simulink model "dspace_2019"  (R2019b)
settings: Solver=FixedStepDiscrete  StartTime=0.0  StopTime=Inf  FixedStep=1e-3  RelTol=1e-3
PostLoadFcn:
  | , if any(exist('dsrtsu_mdlpostloadfcn', 'file') ~= 0), dsrtsu_mdlpostloadfcn('Execute', bdroot); end,
undefined symbols (not defined in the file): ami, amk1_setpoints_1, amk2_setpoints_1, amk3_setpoints_1, amk4_setpoints_1, as, digital, ebs, indicator, mcu_set_dbu_indicator_points, mcu_set_ecu_indicator_points, res_ntm_node_control
libraries: rtican x63, simulink x5, rti1401lib_dio_type3 x4, simulink_extras x1
(part 8 of 16)

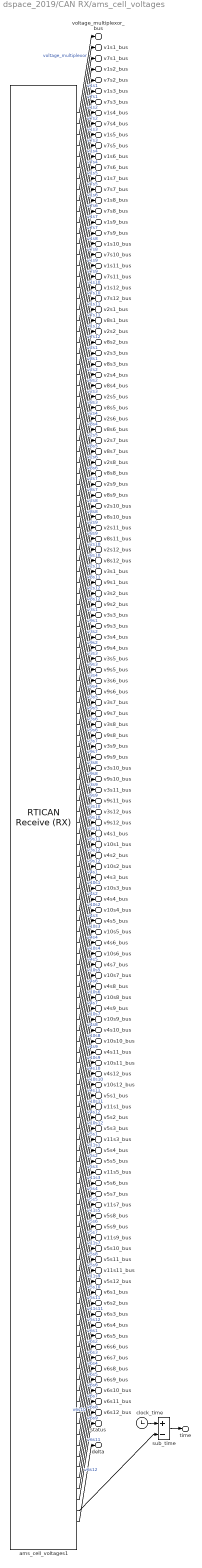
== system dspace_2019/CAN RX/ams_cell_voltages ==
  ams_cell_voltages1 : rtican/RTICAN Receive (RX)   Reserved1=[]  Reserved2=[]  Reserved3=[]  Reserved4=[]  SfcnMessage=[]  Msg_Struct=[]  BoardTypeNo=[]  BoardNo=[]  ChannelNo=[]  Parameters=[]  DialogFcn=[]  UnitName=[]  Revision=[]  UnitValues=[]  DSProperties=struct('RTI',struct('Version',uint32(5),'BlockType',struct('isSLSource',uint8(1),'isSLSink',uint8(1),'isHWSource',uint8(0),'isHWSink',uint8(0),'isSetup',uint8(0),'isInline',uint8(1),'isNonInline',uint8(0),'isInterrupt',uint8(0),'isChannelwise',uint8(0)),'IOBoardType','RTICAN','UnitType','MESSAGE','Identifier','RX','DialogType','MSVC','BlockSet','RTICAN','SlaveProcessor','CAN'))  RTIBlockInterface=struct('OutputPortsWidth',int32([1 1 1 1 1 1 1 1 1 1 1 1 1 1 1 1 1 1 1 1 1 1 1 1 1 1 1 1 1 1 1 1 1 1 1 1 1 1 1 1 1 1 1 1 1 1 1 1 1 1 1 1 1 1 1 1 1 1 1 1 1 1 1 1 1 1 1 1 1 1 1 1 1 1 1 1 1 1 1 1 1 1 1 1 1 1 1 1 1 1 1 1 1 1 1 1 1 1 1 1 1 1 1 1 1 1 1 1 1 1 1 1 1 1 1 1 1 1 1 1 1 1 1 1 1 1 1 1 1 1]),'OutputPortsActive',ones(1,130),'OutputPortsName',{{'voltage_multiplexor','v1s1','v7s1','v1s2','v7s2','v1s3','v7s3','v1s4','v7s4','v1s5','v7s5','v1s6','v7s6','v1s7','v7s7','v1s8','v7s8','v1s9','v7s9','v1s10','v7s10','v1s11','v7s11','v1s12','v7s12','v2s1','v8s1','v2s2','v8s2','v2s3','v8s3','v2s4','v8s4','v2s5','v8s5','v2s6','v8s6','v2s7','v8s7','v2s8','v8s8','v2s9','v8s9','v2s10','v8s10','v2s11','v8s11','v2s12','v8s12','v3s1','v9s1','v3s2','v9s2','v3s3','v9s3','v3s4','v9s4','v3s5','v9s5','v3s6','v9s6','v3s7','v9s7','v3s8','v9s8','v3s9','v9s9','v3s10','v9s10','v3s11','v9s11','v3s12','v9s12','v4s1','v10s1','v4s2','v10s2','v4s3','v10s3','v4s4','v10s4','v4s5','v10s5','v4s6','v10s6','v4s7','v10s7','v4s8','v10s8','v4s9','v10s9','v4s10','v10s10','v4s11','v10s11','v4s12','v10s12','v5s1','v11s1','v5s2','v5s3','v11s3','v5s4','v5s5','v11s5','v5s6','v5s7','v11s7','v5s8','v5s9','v11s9','v5s10','v5s11','v11s11','v5s12','v6s1','v6s2','v6s3','v6s4','v6s5','v6s6','v6s7','v6s8','v6s9','v6s10','v6s11','v6s12',['RX status'],['RX time'],['RX delta time']}},'OutputPortsDataType',{{'SS_DOUBLE','SS_DOUBLE','SS_DOUBLE','SS_DOUBLE','SS_DOUBLE','SS_DOUBLE','SS_DOUBLE','SS_DOUBLE','SS_DOUBLE','SS_DOUBLE','SS_DOUBLE','SS_DOUBLE','SS_DOUBLE','SS_DOUBLE','SS_DOUBLE','SS_DOUBLE','SS_DOUBLE','SS_DOUBLE','SS_DOUBLE','SS_DOUBLE','SS_DOUBLE','SS_DOUBLE','SS_DOUBLE','SS_DOUBLE','SS_DOUBLE','SS_DOUBLE','SS_DOUBLE','SS_DOUBLE','SS_DOUBLE','SS_DOUBLE','SS_DOUBLE','SS_DOUBLE','SS_DOUBLE','SS_DOUBLE','SS_DOUBLE','SS_DOUBLE','SS_DOUBLE','SS_DOUBLE','SS_DOUBLE','SS_DOUBLE','SS_DOUBLE','SS_DOUBLE','SS_DOUBLE','SS_DOUBLE','SS_DOUBLE','SS_DOUBLE','SS_DOUBLE','SS_DOUBLE','SS_DOUBLE','SS_DOUBLE','SS_DOUBLE','SS_DOUBLE','SS_DOUBLE','SS_DOUBLE','SS_DOUBLE','SS_DOUBLE','SS_DOUBLE','SS_DOUBLE','SS_DOUBLE','SS_DOUBLE','SS_DOUBLE','SS_DOUBLE','SS_DOUBLE','SS_DOUBLE','SS_DOUBLE','SS_DOUBLE','SS_DOUBLE','SS_DOUBLE','SS_DOUBLE','SS_DOUBLE','SS_DOUBLE','SS_DOUBLE','SS_DOUBLE','SS_DOUBLE','SS_DOUBLE','SS_DOUBLE','SS_DOUBLE','SS_DOUBLE','SS_DOUBLE','SS_DOUBLE','SS_DOUBLE','SS_DOUBLE','SS_DOUBLE','SS_DOUBLE','SS_DOUBLE','SS_DOUBLE','SS_DOUBLE','SS_DOUBLE','SS_DOUBLE','SS_DOUBLE','SS_DOUBLE','SS_DOUBLE','SS_DOUBLE','SS_DOUBLE','SS_DOUBLE','SS_DOUBLE','SS_DOUBLE','SS_DOUBLE','SS_DOUBLE','SS_DOUBLE','SS_DOUBLE','SS_DOUBLE','SS_DOUBLE','SS_DOUBLE','SS_DOUBLE','SS_DOUBLE','SS_DOUBLE','SS_DOUBLE','SS_DOUBLE','SS_DOUBLE','SS_DOUBLE','SS_DOUBLE','SS_DOUBLE','SS_DOUBLE','SS_DOUBLE','SS_DOUBLE','SS_DOUBLE','SS_DOUBLE','SS_DOUBLE','SS_DOUBLE','SS_DOUBLE','SS_DOUBLE','SS_DOUBLE','SS_DOUBLE','SS_DOUBLE','SS_DOUBLE','SS_DOUBLE','SS_DOUBLE','SS_DOUBLE','SS_DOUBLE'}},'OutputPortsLabel',{{'voltage_multiplexor','v1s1','v7s1','v1s2','v7s2','v1s3','v7s3','v1s4','v7s4','v1s5','v7s5','v1s6','v7s6','v1s7','v7s7','v1s8','v7s8','v1s9','v7s9','v1s10','v7s10','v1s11','v7s11','v1s12','v7s12','v2s1','v8s1','v2s2','v8s2','v2s3','v8s3','v2s4','v8s4','v2s5','v8s5','v2s6','v8s6','v2s7','v8s7','v2s8','v8s8','v2s9','v8s9','v2s10','v8s10','v2s11','v8s11','v2s12','v8s12','v3s1','v9s1','v3s2','v9s2','v3s3','v9s3','v3s4','v9s4','v3s5','v9s5','v3s6','v9s6','v3s7','v9s7','v3s8','v9s8','v3s9','v9s9','v3s10','v9s10','v3s11','v9s11','v3s12','v9s12','v4s1','v10s1','v4s2','v10s2','v4s3','v10s3','v4s4','v10s4','v4s5','v10s5','v4s6','v10s6','v4s7','v10s7','v4s8','v10s8','v4s9','v10s9','v4s10','v10s10','v4s11','v10s11','v4s12','v10s12','v5s1','v11s1','v5s2','v5s3','v11s3','v5s4','v5s5','v11s5','v5s6','v5s7','v11s7','v5s8','v5s9','v11s9','v5s10','v5s11','v11s11','v5s12','v6s1','v6s2','v6s3','v6s4','v6s5','v6s6','v6s7','v6s8','v6s9','v6s10','v6s11','v6s12','','',''}},'OutputPortsLabelMode','ON','InputPortsWidth',int32(0),'InputPortsActive',0,'DialogFcn','rtican_message_interface_gui','BlockDisplay',{{'','center'}},'IconTransparency','on','ParameterTunableNames',{{}},'InitLevel',3,'BlockName',struct('Token',{{'ams_cell_voltages'}}),'SampleTime',{{-1}},'TriggerPort',{{'none'}},'EnablePort',{{'none'}})  RTIBlockParameters=struct('BoardTypeNo',{{1,'OFF',[]}},'BoardNo',{{1,'ON',[1 16]}},'ChannelNo',{{2,'ON',[1 2]}},'Parameters',{{struct('DataFileSupport',struct('DataFileSelectedMaster',1,'DataFileSelectedLocal',1,'DataFileName','c:\users\oscar\documents\github\sw_infrastructure\kthfspe_python\databases\can1.dbc|','DataFileDate',{{{['10-Jul-2022 16:14:04']}}},'SelectedFile','c:\users\oscar\documents\github\sw_infrastructure\kthfspe_python\databases\can1.dbc'),'Options',struct('StatusSelected',1,'TimeSelected',1,'DeltaTimeSelected',1,'BytePortSelected',0,'MessageLengthSelected',0,'TriggerPort',struct('Selected',0,'TriggerType',0),'UserCoding',struct('Selected',0,'InterfaceFile','UserDecodingFile','FcnName','UserDecodeFcn','InportSelected',0,'InportWidth',1,'OutportSelected',0,'OutportWidth',1),'EnablePortSelected',0,'SignalOnPortnameSelected',1,'UseRXService',0),'Message',struct('MsgOnBlocknameSelected',1,'MsgName','ams_cell_voltages','MsgIdFormat',0,'MsgId',33,'MsgLength',7,'NumSignals',127,'SampleTime',-1,'Signal',struct('SgnName',{'voltage_multiplexor','v1s1','v7s1','v1s2','v7s2','v1s3','v7s3','v1s4','v7s4','v1s5','v7s5','v1s6','v7s6','v1s7','v7s7','v1s8','v7s8','v1s9','v7s9','v1s10','v7s10','v1s11','v7s11','v1s12','v7s12','v2s1','v8s1','v2s2','v8s2','v2s3','v8s3','v2s4','v8s4','v2s5','v8s5','v2s6','v8s6','v2s7','v8s7','v2s8','v8s8','v2s9','v8s9','v2s10','v8s10','v2s11','v8s11','v2s12','v8s12','v3s1','v9s1','v3s2','v9s2','v3s3','v9s3','v3s4','v9s4','v3s5','v9s5','v3s6','v9s6','v3s7','v9s7','v3s8','v9s8','v3s9','v9s9','v3s10','v9s10','v3s11','v9s11','v3s12','v9s12','v4s1','v10s1','v4s2','v10s2','v4s3','v10s3','v4s4','v10s4','v4s5','v10s5','v4s6','v10s6','v4s7','v10s7','v4s8','v10s8','v4s9','v10s9','v4s10','v10s10','v4s11','v10s11','v4s12','v10s12','v5s1','v11s1','v5s2','v5s3','v11s3','v5s4','v5s5','v11s5','v5s6','v5s7','v11s7','v5s8','v5s9','v11s9','v5s10','v5s11','v11s11','v5s12','v6s1','v6s2','v6s3','v6s4','v6s5','v6s6','v6s7','v6s8','v6s9','v6s10','v6s11','v6s12'},'SgnStartBit',{0,8,8,8,8,8,8,8,8,8,8,8,8,8,8,8,8,8,8,8,8,8,8,8,8,16,16,16,16,16,16,16,16,16,16,16,16,16,16,16,16,16,16,16,16,16,16,16,16,24,24,24,24,24,24,24,24,24,24,24,24,24,24,24,24,24,24,24,24,24,24,24,24,32,32,32,32,32,32,32,32,32,32,32,32,32,32,32,32,32,32,32,32,32,32,32,32,40,40,40,40,40,40,40,40,40,40,40,40,40,40,40,40,40,40,48,48,48,48,48,48,48,48,48,48,48,48},'SgnLength',{8,8,8,8,8,8,8,8,8,8,8,8,8,8,8,8,8,8,8,8,8,8,8,8,8,8,8,8,8,8,8,8,8,8,8,8,8,8,8,8,8,8,8,8,8,8,8,8,8,8,8,8,8,8,8,8,8,8,8,8,8,8,8,8,8,8,8,8,8,8,8,8,8,8,8,8,8,8,8,8,8,8,8,8,8,8,8,8,8,8,8,8,8,8,8,8,8,8,8,8,8,8,8,8,8,8,8,8,8,8,8,8,8,8,8,8,8,8,8,8,8,8,8,8,8,8,8},'SgnType',{1,2,2,2,2,2,2,2,2,2,2,2,2,2,2,2,2,2,2,2,2,2,2,2,2,2,2,2,2,2,2,2,2,2,2,2,2,2,2,2,2,2,2,2,2,2,2,2,2,2,2,2,2,2,2,2,2,2,2,2,2,2,2,2,2,2,2,2,2,2,2,2,2,2,2,2,2,2,2,2,2,2,2,2,2,2,2,2,2,2,2,2,2,2,2,2,2,2,2,2,2,2,2,2,2,2,2,2,2,2,2,2,2,2,2,2,2,2,2,2,2,2,2,2,2,2,2},'ModeValue',{-1,0,1,2,3,4,5,6,7,8,9,10,11,12,13,14,15,16,17,18,19,20,21,22,23,0,1,2,3,4,5,6,7,8,9,10,11,12,13,14,15,16,17,18,19,20,21,22,23,0,1,2,3,4,5,6,7,8,9,10,11,12,13,14,15,16,17,18,19,20,21,22,23,0,1,2,3,4,5,6,7,8,9,10,11,12,13,14,15,16,17,18,19,20,21,22,23,0,1,2,4,5,6,8,9,10,12,13,14,16,17,18,20,21,22,0,2,4,6,8,10,12,14,16,18,20,22},'DataType',{0,0,0,0,0,0,0,0,0,0,0,0,0,0,0,0,0,0,0,0,0,0,0,0,0,0,0,0,0,0,0,0,0,0,0,0,0,0,0,0,0,0,0,0,0,0,0,0,0,0,0,0,0,0,0,0,0,0,0,0,0,0,0,0,0,0,0,0,0,0,0,0,0,0,0,0,0,0,0,0,0,0,0,0,0,0,0,0,0,0,0,0,0,0,0,0,0,0,0,0,0,0,0,0,0,0,0,0,0,0,0,0,0,0,0,0,0,0,0,0,0,0,0,0,0,0,0},'ByteLayout',{0,0,0,0,0,0,0,0,0,0,0,0,0,0,0,0,0,0,0,0,0,0,0,0,0,0,0,0,0,0,0,0,0,0,0,0,0,0,0,0,0,0,0,0,0,0,0,0,0,0,0,0,0,0,0,0,0,0,0,0,0,0,0,0,0,0,0,0,0,0,0,0,0,0,0,0,0,0,0,0,0,0,0,0,0,0,0,0,0,0,0,0,0,0,0,0,0,0,0,0,0,0,0,0,0,0,0,0,0,0,0,0,0,0,0,0,0,0,0,0,0,0,0,0,0,0,0},'Factor',{1,0.00784,0.00784,0.00784,0.00784,0.00784,0.00784,0.00784,0.00784,0.00784,0.00784,0.00784,0.00784,0.00784,0.00784,0.00784,0.00784,0.00784,0.00784,0.00784,0.00784,0.00784,0.00784,0.00784,0.00784,0.00784,0.00784,0.00784,0.00784,0.00784,0.00784,0.00784,0.00784,0.00784,0.00784,0.00784,0.00784,0.00784,0.00784,0.00784,0.00784,0.00784,0.00784,0.00784,0.00784,0.00784,0.00784,0.00784,0.00784,0.00784,0.00784,0.00784,0.00784,0.00784,0.00784,0.00784,0.00784,0.00784,0.00784,0.00784,0.00784,0.00784,0.00784,0.00784,0.00784,0.00784,0.00784,0.00784,0.00784,0.00784,0.00784,0.00784,0.00784,0.00784,0.00784,0.00784,0.00784,0.00784,0.00784,0.00784,0.00784,0.00784,0.00784,0.00784,0.00784,0.00784,0.00784,0.00784,0.00784,0.00784,0.00784,0.00784,0.00784,0.00784,0.00784,0.00784,0.00784,0.00784,0.00784,0.00784,0.00784,0.00784,0.00784,0.00784,0.00784,0.00784,0.00784,0.00784,0.00784,0.00784,0.00784,0.00784,0.00784,0.00784,0.00784,0.00784,0.00784,0.00784,0.00784,0.00784,0.00784,0.00784,0.00784,0.00784,0.00784,0.00784,0.00784},'Offset',{0,2.5,2.5,2.5,2.5,2.5,2.5,2.5,2.5,2.5,2.5,2.5,2.5,2.5,2.5,2.5,2.5,2.5,2.5,2.5,2.5,2.5,2.5,2.5,2.5,2.5,2.5,2.5,2.5,2.5,2.5,2.5,2.5,2.5,2.5,2.5,2.5,2.5,2.5,2.5,2.5,2.5,2.5,2.5,2.5,2.5,2.5,2.5,2.5,2.5,2.5,2.5,2.5,2.5,2.5,2.5,2.5,2.5,2.5,2.5,2.5,2.5,2.5,2.5,2.5,2.5,2.5,2.5,2.5,2.5,2.5,2.5,2.5,2.5,2.5,2.5,2.5,2.5,2.5,2.5,2.5,2.5,2.5,2.5,2.5,2.5,2.5,2.5,2.5,2.5,2.5,2.5,2.5,2.5,2.5,2.5,2.5,2.5,2.5,2.5,2.5,2.5,2.5,2.5,2.5,2.5,2.5,2.5,2.5,2.5,2.5,2.5,2.5,2.5,2.5,2.5,2.5,2.5,2.5,2.5,2.5,2.5,2.5,2.5,2.5,2.5,2.5},'SgnComment',{{''},{''},{''},{''},{''},{''},{''},{''},{''},{''},{''},{''},{''},{''},{''},{''},{''},{''},{''},{''},{''},{''},{''},{''},{''},{''},{''},{''},{''},{''},{''},{''},{''},{''},{''},{''},{''},{''},{''},{''},{''},{''},{''},{''},{''},{''},{''},{''},{''},{''},{''},{''},{''},{''},{''},{''},{''},{''},{''},{''},{''},{''},{''},{''},{''},{''},{''},{''},{''},{''},{''},{''},{''},{''},{''},{''},{''},{''},{''},{''},{''},{''},{''},{''},{''},{''},{''},{''},{''},{''},{''},{''},{''},{''},{''},{''},{''},{''},{''},{''},{''},{''},{''},{''},{''},{''},{''},{''},{''},{''},{''},{''},{''},{''},{''},{''},{''},{''},{''},{''},{''},{''},{''},{''},{''},{''},{''}},'SgnUnit',{'','V','V','V','V','V','V','V','V','V','V','V','V','V','V','V','V','V','V','V','V','V','V','V','V','V','V','V','V','V','V','V','V','V','V','V','V','V','V','V','V','V','V','V','V','V','V','V','V','V','V','V','V','V','V','V','V','V','V','V','V','V','V','V','V','V','V','V','V','V','V','V','V','V','V','V','V','V','V','V','V','V','V','V','V','V','V','V','V','V','V','V','V','V','V','V','V','V','V','V','V','V','V','V','V','V','V','V','V','V','V','V','V','V','V','V','V','V','V','V','V','V','V','V','V','V','V'},'Min',{0,2.5,2.5,2.5,2.5,2.5,2.5,2.5,2.5,2.5,2.5,2.5,2.5,2.5,2.5,2.5,2.5,2.5,2.5,2.5,2.5,2.5,2.5,2.5,2.5,2.5,2.5,2.5,2.5,2.5,2.5,2.5,2.5,2.5,2.5,2.5,2.5,2.5,2.5,2.5,2.5,2.5,2.5,2.5,2.5,2.5,2.5,2.5,2.5,2.5,2.5,2.5,2.5,2.5,2.5,2.5,2.5,2.5,2.5,2.5,2.5,2.5,2.5,2.5,2.5,2.5,2.5,2.5,2.5,2.5,2.5,2.5,2.5,2.5,2.5,2.5,2.5,2.5,2.5,2.5,2.5,2.5,2.5,2.5,2.5,2.5,2.5,2.5,2.5,2.5,2.5,2.5,2.5,2.5,2.5,2.5,2.5,2.5,2.5,2.5,2.5,2.5,2.5,2.5,2.5,2.5,2.5,2.5,2.5,2.5,2.5,2.5,2.5,2.5,2.5,2.5,2.5,2.5,2.5,2.5,2.5,2.5,2.5,2.5,2.5,2.5,2.5},'Max',{0,4.5,4.5,4.5,4.5,4.5,4.5,4.5,4.5,4.5,4.5,4.5,4.5,4.5,4.5,4.5,4.5,4.5,4.5,4.5,4.5,4.5,4.5,4.5,4.5,4.5,4.5,4.5,4.5,4.5,4.5,4.5,4.5,4.5,4.5,4.5,4.5,4.5,4.5,4.5,4.5,4.5,4.5,4.5,4.5,4.5,4.5,4.5,4.5,4.5,4.5,4.5,4.5,4.5,4.5,4.5,4.5,4.5,4.5,4.5,4.5,4.5,4.5,4.5,4.5,4.5,4.5,4.5,4.5,4.5,4.5,4.5,4.5,4.5,4.5,4.5,4.5,4.5,4.5,4.5,4.5,4.5,4.5,4.5,4.5,4.5,4.5,4.5,4.5,4.5,4.5,4.5,4.5,4.5,4.5,4.5,4.5,4.5,4.5,4.5,4.5,4.5,4.5,4.5,4.5,4.5,4.5,4.5,4.5,4.5,4.5,4.5,4.5,4.5,4.5,4.5,4.5,4.5,4.5,4.5,4.5,4.5,4.5,4.5,4.5,4.5,4.5},'SLDataType',{'SS_DOUBLE','SS_DOUBLE','SS_DOUBLE','SS_DOUBLE','SS_DOUBLE','SS_DOUBLE','SS_DOUBLE','SS_DOUBLE','SS_DOUBLE','SS_DOUBLE','SS_DOUBLE','SS_DOUBLE','SS_DOUBLE','SS_DOUBLE','SS_DOUBLE','SS_DOUBLE','SS_DOUBLE','SS_DOUBLE','SS_DOUBLE','SS_DOUBLE','SS_DOUBLE','SS_DOUBLE','SS_DOUBLE','SS_DOUBLE','SS_DOUBLE','SS_DOUBLE','SS_DOUBLE','SS_DOUBLE','SS_DOUBLE','SS_DOUBLE','SS_DOUBLE','SS_DOUBLE','SS_DOUBLE','SS_DOUBLE','SS_DOUBLE','SS_DOUBLE','SS_DOUBLE','SS_DOUBLE','SS_DOUBLE','SS_DOUBLE','SS_DOUBLE','SS_DOUBLE','SS_DOUBLE','SS_DOUBLE','SS_DOUBLE','SS_DOUBLE','SS_DOUBLE','SS_DOUBLE','SS_DOUBLE','SS_DOUBLE','SS_DOUBLE','SS_DOUBLE','SS_DOUBLE','SS_DOUBLE','SS_DOUBLE','SS_DOUBLE','SS_DOUBLE','SS_DOUBLE','SS_DOUBLE','SS_DOUBLE','SS_DOUBLE','SS_DOUBLE','SS_DOUBLE','SS_DOUBLE','SS_DOUBLE','SS_DOUBLE','SS_DOUBLE','SS_DOUBLE','SS_DOUBLE','SS_DOUBLE','SS_DOUBLE','SS_DOUBLE','SS_DOUBLE','SS_DOUBLE','SS_DOUBLE','SS_DOUBLE','SS_DOUBLE','SS_DOUBLE','SS_DOUBLE','SS_DOUBLE','SS_DOUBLE','SS_DOUBLE','SS_DOUBLE','SS_DOUBLE','SS_DOUBLE','SS_DOUBLE','SS_DOUBLE','SS_DOUBLE','SS_DOUBLE','SS_DOUBLE','SS_DOUBLE','SS_DOUBLE','SS_DOUBLE','SS_DOUBLE','SS_DOUBLE','SS_DOUBLE','SS_DOUBLE','SS_DOUBLE','SS_DOUBLE','SS_DOUBLE','SS_DOUBLE','SS_DOUBLE','SS_DOUBLE','SS_DOUBLE','SS_DOUBLE','SS_DOUBLE','SS_DOUBLE','SS_DOUBLE','SS_DOUBLE','SS_DOUBLE','SS_DOUBLE','SS_DOUBLE','SS_DOUBLE','SS_DOUBLE','SS_DOUBLE','SS_DOUBLE','SS_DOUBLE','SS_DOUBLE','SS_DOUBLE','SS_DOUBLE','SS_DOUBLE','SS_DOUBLE','SS_DOUBLE','SS_DOUBLE','SS_DOUBLE','SS_DOUBLE','SS_DOUBLE'}),'MsgIdNumFormat',0,'MsgComment',{{''}}),'Version',1.2,'general',struct('isFromLib',0)),'OFF',[]}},'GroupId',{{struct('Group',{{'RTICAN'}},'No',1,'Behavior',{{'NAMECHANGE'}},'BlockType',{{'SINK'}},'NameChangeFlag',0),'OFF',[]}},'SFcnRTICANMessage',{{struct('MsgType','RX','SFcnPortType','Scalar','MsgName','ams_cell_voltages','MsgIdFormat','STD','MsgId',33,'MsgLength',7,'NumSignals',127,'SampleTime',-1,'Signal',struct('SgnName',{'voltage_multiplexor','v1s1','v7s1','v1s2','v7s2','v1s3','v7s3','v1s4','v7s4','v1s5','v7s5','v1s6','v7s6','v1s7','v7s7','v1s8','v7s8','v1s9','v7s9','v1s10','v7s10','v1s11','v7s11','v1s12','v7s12','v2s1','v8s1','v2s2','v8s2','v2s3','v8s3','v2s4','v8s4','v2s5','v8s5','v2s6','v8s6','v2s7','v8s7','v2s8','v8s8','v2s9','v8s9','v2s10','v8s10','v2s11','v8s11','v2s12','v8s12','v3s1','v9s1','v3s2','v9s2','v3s3','v9s3','v3s4','v9s4','v3s5','v9s5','v3s6','v9s6','v3s7','v9s7','v3s8','v9s8','v3s9','v9s9','v3s10','v9s10','v3s11','v9s11','v3s12','v9s12','v4s1','v10s1','v4s2','v10s2','v4s3','v10s3','v4s4','v10s4','v4s5','v10s5','v4s6','v10s6','v4s7','v10s7','v4s8','v10s8','v4s9','v10s9','v4s10','v10s10','v4s11','v10s11','v4s12','v10s12','v5s1','v11s1','v5s2','v5s3','v11s3','v5s4','v5s5','v11s5','v5s6','v5s7','v11s7','v5s8','v5s9','v11s9','v5s10','v5s11','v11s11','v5s12','v6s1','v6s2','v6s3','v6s4','v6s5','v6s6','v6s7','v6s8','v6s9','v6s10','v6s11','v6s12'},'SgnStartBit',{0,8,8,8,8,8,8,8,8,8,8,8,8,8,8,8,8,8,8,8,8,8,8,8,8,16,16,16,16,16,16,16,16,16,16,16,16,16,16,16,16,16,16,16,16,16,16,16,16,24,24,24,24,24,24,24,24,24,24,24,24,24,24,24,24,24,24,24,24,24,24,24,24,32,32,32,32,32,32,32,32,32,32,32,32,32,32,32,32,32,32,32,32,32,32,32,32,40,40,40,40,40,40,40,40,40,40,40,40,40,40,40,40,40,40,48,48,48,48,48,48,48,48,48,48,48,48},'SgnLength',{8,8,8,8,8,8,8,8,8,8,8,8,8,8,8,8,8,8,8,8,8,8,8,8,8,8,8,8,8,8,8,8,8,8,8,8,8,8,8,8,8,8,8,8,8,8,8,8,8,8,8,8,8,8,8,8,8,8,8,8,8,8,8,8,8,8,8,8,8,8,8,8,8,8,8,8,8,8,8,8,8,8,8,8,8,8,8,8,8,8,8,8,8,8,8,8,8,8,8,8,8,8,8,8,8,8,8,8,8,8,8,8,8,8,8,8,8,8,8,8,8,8,8,8,8,8,8},'SgnType',{'mode','mode-dependent','mode-dependent','mode-dependent','mode-dependent','mode-dependent','mode-dependent','mode-dependent','mode-dependent','mode-dependent','mode-dependent','mode-dependent','mode-dependent','mode-dependent','mode-dependent','mode-dependent','mode-dependent','mode-dependent','mode-dependent','mode-dependent','mode-dependent','mode-dependent','mode-dependent','mode-dependent','mode-dependent','mode-dependent','mode-dependent','mode-dependent','mode-dependent','mode-dependent','mode-dependent','mode-dependent','mode-dependent','mode-dependent','mode-dependent','mode-dependent','mode-dependent','mode-dependent','mode-dependent','mode-dependent','mode-dependent','mode-dependent','mode-dependent','mode-dependent','mode-dependent','mode-dependent','mode-dependent','mode-dependent','mode-dependent','mode-dependent','mode-dependent','mode-dependent','mode-dependent','mode-dependent','mode-dependent','mode-dependent','mode-dependent','mode-dependent','mode-dependent','mode-dependent','mode-dependent','mode-dependent','mode-dependent','mode-dependent','mode-dependent','mode-dependent','mode-dependent','mode-dependent','mode-dependent','mode-dependent','mode-dependent','mode-dependent','mode-dependent','mode-dependent','mode-dependent','mode-dependent','mode-dependent','mode-dependent','mode-dependent','mode-dependent','mode-dependent','mode-dependent','mode-dependent','mode-dependent','mode-dependent','mode-dependent','mode-dependent','mode-dependent','mode-dependent','mode-dependent','mode-dependent','mode-dependent','mode-dependent','mode-dependent','mode-dependent','mode-dependent','mode-dependent','mode-dependent','mode-dependent','mode-dependent','mode-dependent','mode-dependent','mode-dependent','mode-dependent','mode-dependent','mode-dependent','mode-dependent','mode-dependent','mode-dependent','mode-dependent','mode-dependent','mode-dependent','mode-dependent','mode-dependent','mode-dependent','mode-dependent','mode-dependent','mode-dependent','mode-dependent','mode-dependent','mode-dependent','mode-dependent','mode-dependent','mode-dependent','mode-dependent','mode-dependent','mode-dependent'},'ModeValue',{-1,0,1,2,3,4,5,6,7,8,9,10,11,12,13,14,15,16,17,18,19,20,21,22,23,0,1,2,3,4,5,6,7,8,9,10,11,12,13,14,15,16,17,18,19,20,21,22,23,0,1,2,3,4,5,6,7,8,9,10,11,12,13,14,15,16,17,18,19,20,21,22,23,0,1,2,3,4,5,6,7,8,9,10,11,12,13,14,15,16,17,18,19,20,21,22,23,0,1,2,4,5,6,8,9,10,12,13,14,16,17,18,20,21,22,0,2,4,6,8,10,12,14,16,18,20,22},'DataType',{['unsigned int'],['unsigned int'],['unsigned int'],['unsigned int'],['unsigned int'],['unsigned int'],['unsigned int'],['unsigned int'],['unsigned int'],['unsigned int'],['unsigned int'],['unsigned int'],['unsigned int'],['unsigned int'],['unsigned int'],['unsigned int'],['unsigned int'],['unsigned int'],['unsigned int'],['unsigned int'],['unsigned int'],['unsigned int'],['unsigned int'],['unsigned int'],['unsigned int'],['unsigned int'],['unsigned int'],['unsigned int'],['unsigned int'],['unsigned int'],['unsigned int'],['unsigned int'],['unsigned int'],['unsigned int'],['unsigned int'],['unsigned int'],['unsigned int'],['unsigned int'],['unsigned int'],['unsigned int'],['unsigned int'],['unsigned int'],['unsigned int'],['unsigned int'],['unsigned int'],['unsigned int'],['unsigned int'],['unsigned int'],['unsigned int'],['unsigned int'],['unsigned int'],['unsigned int'],['unsigned int'],['unsigned int'],['unsigned int'],['unsigned int'],['unsigned int'],['unsigned int'],['unsigned int'],['unsigned int'],['unsigned int'],['unsigned int'],['unsigned int'],['unsigned int'],['unsigned int'],['unsigned int'],['unsigned int'],['unsigned int'],['unsigned int'],['unsigned int'],['unsigned int'],['unsigned int'],['unsigned int'],['unsigned int'],['unsigned int'],['unsigned int'],['unsigned int'],['unsigned int'],['unsigned int'],['unsigned int'],['unsigned int'],['unsigned int'],['unsigned int'],['unsigned int'],['unsigned int'],['unsigned int'],['unsigned int'],['unsigned int'],['unsigned int'],['unsigned int'],['unsigned int'],['unsigned int'],['unsigned int'],['unsigned int'],['unsigned int'],['unsigned int'],['unsigned int'],['unsigned int'],['unsigned int'],['unsigned int'],['unsigned int'],['unsigned int'],['unsigned int'],['unsigned int'],['unsigned int'],['unsigned int'],['unsigned int'],['unsigned int'],['unsigned int'],['unsigned int'],['unsigned int'],['unsigned int'],['unsigned int'],['unsigned int'],['unsigned int'],['unsigned int'],['unsigned int'],['unsigned int'],['unsigned int'],['unsigned int'],['unsigned int'],['unsigned int'],['unsigned int'],['unsigned int'],['unsigned int'],['unsigned int'],['unsigned int']},'ByteLayout',{['little endian'],['little endian'],['little endian'],['little endian'],['little endian'],['little endian'],['little endian'],['little endian'],['little endian'],['little endian'],['little endian'],['little endian'],['little endian'],['little endian'],['little endian'],['little endian'],['little endian'],['little endian'],['little endian'],['little endian'],['little endian'],['little endian'],['little endian'],['little endian'],['little endian'],['little endian'],['little endian'],['little endian'],['little endian'],['little endian'],['little endian'],['little endian'],['little endian'],['little endian'],['little endian'],['little endian'],['little endian'],['little endian'],['little endian'],['little endian'],['little endian'],['little endian'],['little endian'],['little endian'],['little endian'],['little endian'],['little endian'],['little endian'],['little endian'],['little endian'],['little endian'],['little endian'],['little endian'],['little endian'],['little endian'],['little endian'],['little endian'],['little endian'],['little endian'],['little endian'],['little endian'],['little endian'],['little endian'],['little endian'],['little endian'],['little endian'],['little endian'],['little endian'],['little endian'],['little endian'],['little endian'],['little endian'],['little endian'],['little endian'],['little endian'],['little endian'],['little endian'],['little endian'],['little endian'],['little endian'],['little endian'],['little endian'],['little endian'],['little endian'],['little endian'],['little endian'],['little endian'],['little endian'],['little endian'],['little endian'],['little endian'],['little endian'],['little endian'],['little endian'],['little endian'],['little endian'],['little endian'],['little endian'],['little endian'],['little endian'],['little endian'],['little endian'],['little endian'],['little endian'],['little endian'],['little endian'],['little endian'],['little endian'],['little endian'],['little endian'],['little endian'],['little endian'],['little endian'],['little endian'],['little endian'],['little endian'],['little endian'],['little endian'],['little endian'],['little endian'],['little endian'],['little endian'],['little endian'],['little endian'],['little endian'],['little endian'],['little endian']},'Factor',{1,0.00784,0.00784,0.00784,0.00784,0.00784,0.00784,0.00784,0.00784,0.00784,0.00784,0.00784,0.00784,0.00784,0.00784,0.00784,0.00784,0.00784,0.00784,0.00784,0.00784,0.00784,0.00784,0.00784,0.00784,0.00784,0.00784,0.00784,0.00784,0.00784,0.00784,0.00784,0.00784,0.00784,0.00784,0.00784,0.00784,0.00784,0.00784,0.00784,0.00784,0.00784,0.00784,0.00784,0.00784,0.00784,0.00784,0.00784,0.00784,0.00784,0.00784,0.00784,0.00784,0.00784,0.00784,0.00784,0.00784,0.00784,0.00784,0.00784,0.00784,0.00784,0.00784,0.00784,0.00784,0.00784,0.00784,0.00784,0.00784,0.00784,0.00784,0.00784,0.00784,0.00784,0.00784,0.00784,0.00784,0.00784,0.00784,0.00784,0.00784,0.00784,0.00784,0.00784,0.00784,0.00784,0.00784,0.00784,0.00784,0.00784,0.00784,0.00784,0.00784,0.00784,0.00784,0.00784,0.00784,0.00784,0.00784,0.00784,0.00784,0.00784,0.00784,0.00784,0.00784,0.00784,0.00784,0.00784,0.00784,0.00784,0.00784,0.00784,0.00784,0.00784,0.00784,0.00784,0.00784,0.00784,0.00784,0.00784,0.00784,0.00784,0.00784,0.00784,0.00784,0.00784,0.00784},'Offset',{0,2.5,2.5,2.5,2.5,2.5,2.5,2.5,2.5,2.5,2.5,2.5,2.5,2.5,2.5,2.5,2.5,2.5,2.5,2.5,2.5,2.5,2.5,2.5,2.5,2.5,2.5,2.5,2.5,2.5,2.5,2.5,2.5,2.5,2.5,2.5,2.5,2.5,2.5,2.5,2.5,2.5,2.5,2.5,2.5,2.5,2.5,2.5,2.5,2.5,2.5,2.5,2.5,2.5,2.5,2.5,2.5,2.5,2.5,2.5,2.5,2.5,2.5,2.5,2.5,2.5,2.5,2.5,2.5,2.5,2.5,2.5,2.5,2.5,2.5,2.5,2.5,2.5,2.5,2.5,2.5,2.5,2.5,2.5,2.5,2.5,2.5,2.5,2.5,2.5,2.5,2.5,2.5,2.5,2.5,2.5,2.5,2.5,2.5,2.5,2.5,2.5,2.5,2.5,2.5,2.5,2.5,2.5,2.5,2.5,2.5,2.5,2.5,2.5,2.5,2.5,2.5,2.5,2.5,2.5,2.5,2.5,2.5,2.5,2.5,2.5,2.5},'SLDataType',{'SS_DOUBLE','SS_DOUBLE','SS_DOUBLE','SS_DOUBLE','SS_DOUBLE','SS_DOUBLE','SS_DOUBLE','SS_DOUBLE','SS_DOUBLE','SS_DOUBLE','SS_DOUBLE','SS_DOUBLE','SS_DOUBLE','SS_DOUBLE','SS_DOUBLE','SS_DOUBLE','SS_DOUBLE','SS_DOUBLE','SS_DOUBLE','SS_DOUBLE','SS_DOUBLE','SS_DOUBLE','SS_DOUBLE','SS_DOUBLE','SS_DOUBLE','SS_DOUBLE','SS_DOUBLE','SS_DOUBLE','SS_DOUBLE','SS_DOUBLE','SS_DOUBLE','SS_DOUBLE','SS_DOUBLE','SS_DOUBLE','SS_DOUBLE','SS_DOUBLE','SS_DOUBLE','SS_DOUBLE','SS_DOUBLE','SS_DOUBLE','SS_DOUBLE','SS_DOUBLE','SS_DOUBLE','SS_DOUBLE','SS_DOUBLE','SS_DOUBLE','SS_DOUBLE','SS_DOUBLE','SS_DOUBLE','SS_DOUBLE','SS_DOUBLE','SS_DOUBLE','SS_DOUBLE','SS_DOUBLE','SS_DOUBLE','SS_DOUBLE','SS_DOUBLE','SS_DOUBLE','SS_DOUBLE','SS_DOUBLE','SS_DOUBLE','SS_DOUBLE','SS_DOUBLE','SS_DOUBLE','SS_DOUBLE','SS_DOUBLE','SS_DOUBLE','SS_DOUBLE','SS_DOUBLE','SS_DOUBLE','SS_DOUBLE','SS_DOUBLE','SS_DOUBLE','SS_DOUBLE','SS_DOUBLE','SS_DOUBLE','SS_DOUBLE','SS_DOUBLE','SS_DOUBLE','SS_DOUBLE','SS_DOUBLE','SS_DOUBLE','SS_DOUBLE','SS_DOUBLE','SS_DOUBLE','SS_DOUBLE','SS_DOUBLE','SS_DOUBLE','SS_DOUBLE','SS_DOUBLE','SS_DOUBLE','SS_DOUBLE','SS_DOUBLE','SS_DOUBLE','SS_DOUBLE','SS_DOUBLE','SS_DOUBLE','SS_DOUBLE','SS_DOUBLE','SS_DOUBLE','SS_DOUBLE','SS_DOUBLE','SS_DOUBLE','SS_DOUBLE','SS_DOUBLE','SS_DOUBLE','SS_DOUBLE','SS_DOUBLE','SS_DOUBLE','SS_DOUBLE','SS_DOUBLE','SS_DOUBLE','SS_DOUBLE','SS_DOUBLE','SS_DOUBLE','SS_DOUBLE','SS_DOUBLE','SS_DOUBLE','SS_DOUBLE','SS_DOUBLE','SS_DOUBLE','SS_DOUBLE','SS_DOUBLE','SS_DOUBLE','SS_DOUBLE','SS_DOUBLE','SS_DOUBLE'}),'StatusSelected','yes','TimeSelected','yes','DeltaTimeSelected','yes','BytePortSelected','no','MessageLengthSelected','no','TriggerPort',struct('Selected','no','TriggerType',0),'UserCoding',struct('Selected','no','InterfaceFile','UserDecodingFile','FcnName','UserDecodeFcn','InportSelected','no','InportWidth',1,'OutportSelected','no','OutportWidth',1),'EnablePortSelected','no','UseRXService','no','BoardType','DS1','BoardNo',1,'ControllerNo',1),'OFF',[]}},'TLCFileName',{{'rtican_rx_message','OFF',[]}})  RTISFcnParameters=struct('SFcnRTICANMessage','struct','TLCFileName','char')  RTIBlockParaDefault=struct('BoardTypeNo',4302,'BoardNo',1,'ChannelNo',1,'Parameters',struct('DataFileSupport',struct('DataFileSelectedMaster',0,'DataFileSelectedLocal',0,'DataFileName','','DataFileDate','','SelectedFile',['<no file selected>']),'Options',struct('StatusSelected',1,'TimeSelected',1,'DeltaTimeSelected',1,'BytePortSelected',0,'MessageLengthSelected',0,'TriggerPort',struct('Selected',0,'TriggerType','rising'),'UserCoding',struct('Selected',0,'InterfaceFile','UserDecodingFile','FcnName','UserDecodeFcn','InportSelected',0,'InportWidth',1,'OutportSelected',0,'OutportWidth',1),'EnablePortSelected',0,'SignalOnPortnameSelected',1,'UseRXService',0),'Message',struct('MsgOnBlocknameSelected',0,'MsgName',['RX Message'],'MsgIdFormat',0,'MsgId',100,'MsgLength',8,'NumSignals',1,'SampleTime',-1,'Signal',struct('SgnName',['RX signal'],'SgnStartBit',0,'SgnLength',8,'SgnType',0,'ModeValue',-1,'DataType',0,'SLDataType','SS_DOUBLE','ByteLayout',0,'Factor',1,'Offset',0,'Min',0,'Max',255,'SgnComment',{{}},'SgnUnit',''),'MsgIdNumFormat',0,'MsgComment',{{''}}),'Version',1.2,'general',struct('isFromLib',1)),'GroupId',struct('Group',{{'RTICAN'}},'No',1,'Behavior',{{'NAMECHANGE'}},'BlockType',{{'SINK'}},'NameChangeFlag',0),'SFcnRTICANMessage',struct('MsgType','RX','MsgName',['RX Message'],'MsgIdFormat','STD','MsgId',100,'MsgLength',8,'NumSignals',1,'SampleTime',-1,'Signal',struct('SgnName',['RX signal'],'SgnStartBit',0,'SgnLength',8,'SgnType','standard','ModeValue',-1,'DataType',['unsigned int'],'ByteLayout',['little endian'],'SLDataType','SS_DOUBLE','Factor',1,'Offset',0),'StatusSelected','yes','TimeSelected','yes','DeltaTimeSelected','yes','BytePortSelected','no','MessageLengthSelected','no','EnablePortSelected','no','UserCoding',struct('Selected','no','InterfaceFile','UserDecodingFile','FcnName','UserDecodeFcn','InportSelected','no','InportWidth',1,'OutportSelected','no','OutportWidth',1),'TriggerPort',struct('Selected','no','TriggerType','rising'),'UseRXService','no','BoardType','DS4302','BoardNo',1,'ControllerNo',1,'SFcnPortType','Scalar'),'TLCFileName','rtican_rx_message')
      settings: AttributesFormatString=Group Id: RTICAN1\n  SourceProductName=dSPACE RTI CAN Blockset
  clock_time : Clock
  sub_time : Sum  Inputs=+-
  voltage_multiplexor_bus : Outport  PortName=signals  Element=voltage_multiplexor
  v1s1_bus : Outport  PortName=signals  Element=v1s1
  v7s1_bus : Outport  PortName=signals  Element=v7s1
  v1s2_bus : Outport  PortName=signals  Element=v1s2
  v7s2_bus : Outport  PortName=signals  Element=v7s2
  v1s3_bus : Outport  PortName=signals  Element=v1s3
  v7s3_bus : Outport  PortName=signals  Element=v7s3
  v1s4_bus : Outport  PortName=signals  Element=v1s4
  v7s4_bus : Outport  PortName=signals  Element=v7s4
  v1s5_bus : Outport  PortName=signals  Element=v1s5
  v7s5_bus : Outport  PortName=signals  Element=v7s5
  v1s6_bus : Outport  PortName=signals  Element=v1s6
  v7s6_bus : Outport  PortName=signals  Element=v7s6
  v1s7_bus : Outport  PortName=signals  Element=v1s7
  v7s7_bus : Outport  PortName=signals  Element=v7s7
  v1s8_bus : Outport  PortName=signals  Element=v1s8
  v7s8_bus : Outport  PortName=signals  Element=v7s8
  v1s9_bus : Outport  PortName=signals  Element=v1s9
  v7s9_bus : Outport  PortName=signals  Element=v7s9
  v1s10_bus : Outport  PortName=signals  Element=v1s10
  v7s10_bus : Outport  PortName=signals  Element=v7s10
  v1s11_bus : Outport  PortName=signals  Element=v1s11
  v7s11_bus : Outport  PortName=signals  Element=v7s11
  v1s12_bus : Outport  PortName=signals  Element=v1s12
  v7s12_bus : Outport  PortName=signals  Element=v7s12
  v2s1_bus : Outport  PortName=signals  Element=v2s1
  v8s1_bus : Outport  PortName=signals  Element=v8s1
  v2s2_bus : Outport  PortName=signals  Element=v2s2
  v8s2_bus : Outport  PortName=signals  Element=v8s2
  v2s3_bus : Outport  PortName=signals  Element=v2s3
  v8s3_bus : Outport  PortName=signals  Element=v8s3
  v2s4_bus : Outport  PortName=signals  Element=v2s4
  v8s4_bus : Outport  PortName=signals  Element=v8s4
  v2s5_bus : Outport  PortName=signals  Element=v2s5
  v8s5_bus : Outport  PortName=signals  Element=v8s5
  v2s6_bus : Outport  PortName=signals  Element=v2s6
  v8s6_bus : Outport  PortName=signals  Element=v8s6
  v2s7_bus : Outport  PortName=signals  Element=v2s7
  v8s7_bus : Outport  PortName=signals  Element=v8s7
  v2s8_bus : Outport  PortName=signals  Element=v2s8
  v8s8_bus : Outport  PortName=signals  Element=v8s8
  v2s9_bus : Outport  PortName=signals  Element=v2s9
  v8s9_bus : Outport  PortName=signals  Element=v8s9
  v2s10_bus : Outport  PortName=signals  Element=v2s10
  v8s10_bus : Outport  PortName=signals  Element=v8s10
  v2s11_bus : Outport  PortName=signals  Element=v2s11
  v8s11_bus : Outport  PortName=signals  Element=v8s11
  v2s12_bus : Outport  PortName=signals  Element=v2s12
  v8s12_bus : Outport  PortName=signals  Element=v8s12
  v3s1_bus : Outport  PortName=signals  Element=v3s1
  v9s1_bus : Outport  PortName=signals  Element=v9s1
  v3s2_bus : Outport  PortName=signals  Element=v3s2
  v9s2_bus : Outport  PortName=signals  Element=v9s2
  v3s3_bus : Outport  PortName=signals  Element=v3s3
  v9s3_bus : Outport  PortName=signals  Element=v9s3
  v3s4_bus : Outport  PortName=signals  Element=v3s4
  v9s4_bus : Outport  PortName=signals  Element=v9s4
  v3s5_bus : Outport  PortName=signals  Element=v3s5
  v9s5_bus : Outport  PortName=signals  Element=v9s5
  v3s6_bus : Outport  PortName=signals  Element=v3s6
  v9s6_bus : Outport  PortName=signals  Element=v9s6
  v3s7_bus : Outport  PortName=signals  Element=v3s7
  v9s7_bus : Outport  PortName=signals  Element=v9s7
  v3s8_bus : Outport  PortName=signals  Element=v3s8
  v9s8_bus : Outport  PortName=signals  Element=v9s8
  v3s9_bus : Outport  PortName=signals  Element=v3s9
  v9s9_bus : Outport  PortName=signals  Element=v9s9
  v3s10_bus : Outport  PortName=signals  Element=v3s10
  v9s10_bus : Outport  PortName=signals  Element=v9s10
  v3s11_bus : Outport  PortName=signals  Element=v3s11
  v9s11_bus : Outport  PortName=signals  Element=v9s11
  v3s12_bus : Outport  PortName=signals  Element=v3s12
  v9s12_bus : Outport  PortName=signals  Element=v9s12
  v4s1_bus : Outport  PortName=signals  Element=v4s1
  v10s1_bus : Outport  PortName=signals  Element=v10s1
  v4s2_bus : Outport  PortName=signals  Element=v4s2
  v10s2_bus : Outport  PortName=signals  Element=v10s2
  v4s3_bus : Outport  PortName=signals  Element=v4s3
  v10s3_bus : Outport  PortName=signals  Element=v10s3
  v4s4_bus : Outport  PortName=signals  Element=v4s4
  v10s4_bus : Outport  PortName=signals  Element=v10s4
  v4s5_bus : Outport  PortName=signals  Element=v4s5
  v10s5_bus : Outport  PortName=signals  Element=v10s5
  v4s6_bus : Outport  PortName=signals  Element=v4s6
  v10s6_bus : Outport  PortName=signals  Element=v10s6
  v4s7_bus : Outport  PortName=signals  Element=v4s7
  v10s7_bus : Outport  PortName=signals  Element=v10s7
  v4s8_bus : Outport  PortName=signals  Element=v4s8
  v10s8_bus : Outport  PortName=signals  Element=v10s8
  v4s9_bus : Outport  PortName=signals  Element=v4s9
  v10s9_bus : Outport  PortName=signals  Element=v10s9
  v4s10_bus : Outport  PortName=signals  Element=v4s10
  v10s10_bus : Outport  PortName=signals  Element=v10s10
  v4s11_bus : Outport  PortName=signals  Element=v4s11
  v10s11_bus : Outport  PortName=signals  Element=v10s11
  v4s12_bus : Outport  PortName=signals  Element=v4s12
  v10s12_bus : Outport  PortName=signals  Element=v10s12
  v5s1_bus : Outport  PortName=signals  Element=v5s1
  v11s1_bus : Outport  PortName=signals  Element=v11s1
  v5s2_bus : Outport  PortName=signals  Element=v5s2
  v5s3_bus : Outport  PortName=signals  Element=v5s3
  v11s3_bus : Outport  PortName=signals  Element=v11s3
  v5s4_bus : Outport  PortName=signals  Element=v5s4
  v5s5_bus : Outport  PortName=signals  Element=v5s5
  v11s5_bus : Outport  PortName=signals  Element=v11s5
  v5s6_bus : Outport  PortName=signals  Element=v5s6
  v5s7_bus : Outport  PortName=signals  Element=v5s7
  v11s7_bus : Outport  PortName=signals  Element=v11s7
  v5s8_bus : Outport  PortName=signals  Element=v5s8
  v5s9_bus : Outport  PortName=signals  Element=v5s9
  v11s9_bus : Outport  PortName=signals  Element=v11s9
  v5s10_bus : Outport  PortName=signals  Element=v5s10
  v5s11_bus : Outport  PortName=signals  Element=v5s11
  v11s11_bus : Outport  PortName=signals  Element=v11s11
  v5s12_bus : Outport  PortName=signals  Element=v5s12
  v6s1_bus : Outport  PortName=signals  Element=v6s1
  v6s2_bus : Outport  PortName=signals  Element=v6s2
  v6s3_bus : Outport  PortName=signals  Element=v6s3
  v6s4_bus : Outport  PortName=signals  Element=v6s4
  v6s5_bus : Outport  PortName=signals  Element=v6s5
  v6s6_bus : Outport  PortName=signals  Element=v6s6
  v6s7_bus : Outport  PortName=signals  Element=v6s7
  v6s8_bus : Outport  PortName=signals  Element=v6s8
  v6s9_bus : Outport  PortName=signals  Element=v6s9
  v6s10_bus : Outport  PortName=signals  Element=v6s10
  v6s11_bus : Outport  PortName=signals  Element=v6s11
  v6s12_bus : Outport  PortName=signals  Element=v6s12
  status : Outport  Port=2
  time : Outport  Port=3
  delta : Outport  Port=4
  wires:
  clock_time/1 -> sub_time/1
  sub_time/1 -> time/1
  ams_cell_voltages1/128 -> status/1
  ams_cell_voltages1/129 -> sub_time/2
  ams_cell_voltages1/130 -> delta/1
  ams_cell_voltages1/1 -> voltage_multiplexor_bus/1  "voltage_multiplexor"
  ams_cell_voltages1/2 -> v1s1_bus/1  "v1s1"
  ams_cell_voltages1/3 -> v7s1_bus/1  "v7s1"
  ams_cell_voltages1/4 -> v1s2_bus/1  "v1s2"
  ams_cell_voltages1/5 -> v7s2_bus/1  "v7s2"
  ams_cell_voltages1/6 -> v1s3_bus/1  "v1s3"
  ams_cell_voltages1/7 -> v7s3_bus/1  "v7s3"
  ams_cell_voltages1/8 -> v1s4_bus/1  "v1s4"
  ams_cell_voltages1/9 -> v7s4_bus/1  "v7s4"
  ams_cell_voltages1/10 -> v1s5_bus/1  "v1s5"
  ams_cell_voltages1/11 -> v7s5_bus/1  "v7s5"
  ams_cell_voltages1/12 -> v1s6_bus/1  "v1s6"
  ams_cell_voltages1/13 -> v7s6_bus/1  "v7s6"
  ams_cell_voltages1/14 -> v1s7_bus/1  "v1s7"
  ams_cell_voltages1/15 -> v7s7_bus/1  "v7s7"
  ams_cell_voltages1/16 -> v1s8_bus/1  "v1s8"
  ams_cell_voltages1/17 -> v7s8_bus/1  "v7s8"
  ams_cell_voltages1/18 -> v1s9_bus/1  "v1s9"
  ams_cell_voltages1/19 -> v7s9_bus/1  "v7s9"
  ams_cell_voltages1/20 -> v1s10_bus/1  "v1s10"
  ams_cell_voltages1/21 -> v7s10_bus/1  "v7s10"
  ams_cell_voltages1/22 -> v1s11_bus/1  "v1s11"
  ams_cell_voltages1/23 -> v7s11_bus/1  "v7s11"
  ams_cell_voltages1/24 -> v1s12_bus/1  "v1s12"
  ams_cell_voltages1/25 -> v7s12_bus/1  "v7s12"
  ams_cell_voltages1/26 -> v2s1_bus/1  "v2s1"
  ams_cell_voltages1/27 -> v8s1_bus/1  "v8s1"
  ams_cell_voltages1/28 -> v2s2_bus/1  "v2s2"
  ams_cell_voltages1/29 -> v8s2_bus/1  "v8s2"
  ams_cell_voltages1/30 -> v2s3_bus/1  "v2s3"
  ams_cell_voltages1/31 -> v8s3_bus/1  "v8s3"
  ams_cell_voltages1/32 -> v2s4_bus/1  "v2s4"
  ams_cell_voltages1/33 -> v8s4_bus/1  "v8s4"
  ams_cell_voltages1/34 -> v2s5_bus/1  "v2s5"
  ams_cell_voltages1/35 -> v8s5_bus/1  "v8s5"
  ams_cell_voltages1/36 -> v2s6_bus/1  "v2s6"
  ams_cell_voltages1/37 -> v8s6_bus/1  "v8s6"
  ams_cell_voltages1/38 -> v2s7_bus/1  "v2s7"
  ams_cell_voltages1/39 -> v8s7_bus/1  "v8s7"
  ams_cell_voltages1/40 -> v2s8_bus/1  "v2s8"
  ams_cell_voltages1/41 -> v8s8_bus/1  "v8s8"
  ams_cell_voltages1/42 -> v2s9_bus/1  "v2s9"
  ams_cell_voltages1/43 -> v8s9_bus/1  "v8s9"
  ams_cell_voltages1/44 -> v2s10_bus/1  "v2s10"
  ams_cell_voltages1/45 -> v8s10_bus/1  "v8s10"
  ams_cell_voltages1/46 -> v2s11_bus/1  "v2s11"
  ams_cell_voltages1/47 -> v8s11_bus/1  "v8s11"
  ams_cell_voltages1/48 -> v2s12_bus/1  "v2s12"
  ams_cell_voltages1/49 -> v8s12_bus/1  "v8s12"
  ams_cell_voltages1/50 -> v3s1_bus/1  "v3s1"
  ams_cell_voltages1/51 -> v9s1_bus/1  "v9s1"
  ams_cell_voltages1/52 -> v3s2_bus/1  "v3s2"
  ams_cell_voltages1/53 -> v9s2_bus/1  "v9s2"
  ams_cell_voltages1/54 -> v3s3_bus/1  "v3s3"
  ams_cell_voltages1/55 -> v9s3_bus/1  "v9s3"
  ams_cell_voltages1/56 -> v3s4_bus/1  "v3s4"
  ams_cell_voltages1/57 -> v9s4_bus/1  "v9s4"
  ams_cell_voltages1/58 -> v3s5_bus/1  "v3s5"
  ams_cell_voltages1/59 -> v9s5_bus/1  "v9s5"
  ams_cell_voltages1/60 -> v3s6_bus/1  "v3s6"
  ams_cell_voltages1/61 -> v9s6_bus/1  "v9s6"
  ams_cell_voltages1/62 -> v3s7_bus/1  "v3s7"
  ams_cell_voltages1/63 -> v9s7_bus/1  "v9s7"
  ams_cell_voltages1/64 -> v3s8_bus/1  "v3s8"
  ams_cell_voltages1/65 -> v9s8_bus/1  "v9s8"
  ams_cell_voltages1/66 -> v3s9_bus/1  "v3s9"
  ams_cell_voltages1/67 -> v9s9_bus/1  "v9s9"
  ams_cell_voltages1/68 -> v3s10_bus/1  "v3s10"
  ams_cell_voltages1/69 -> v9s10_bus/1  "v9s10"
  ams_cell_voltages1/70 -> v3s11_bus/1  "v3s11"
  ams_cell_voltages1/71 -> v9s11_bus/1  "v9s11"
  ams_cell_voltages1/72 -> v3s12_bus/1  "v3s12"
  ams_cell_voltages1/73 -> v9s12_bus/1  "v9s12"
  ams_cell_voltages1/74 -> v4s1_bus/1  "v4s1"
  ams_cell_voltages1/75 -> v10s1_bus/1  "v10s1"
  ams_cell_voltages1/76 -> v4s2_bus/1  "v4s2"
  ams_cell_voltages1/77 -> v10s2_bus/1  "v10s2"
  ams_cell_voltages1/78 -> v4s3_bus/1  "v4s3"
  ams_cell_voltages1/79 -> v10s3_bus/1  "v10s3"
  ams_cell_voltages1/80 -> v4s4_bus/1  "v4s4"
  ams_cell_voltages1/81 -> v10s4_bus/1  "v10s4"
  ams_cell_voltages1/82 -> v4s5_bus/1  "v4s5"
  ams_cell_voltages1/83 -> v10s5_bus/1  "v10s5"
  ams_cell_voltages1/84 -> v4s6_bus/1  "v4s6"
  ams_cell_voltages1/85 -> v10s6_bus/1  "v10s6"
  ams_cell_voltages1/86 -> v4s7_bus/1  "v4s7"
  ams_cell_voltages1/87 -> v10s7_bus/1  "v10s7"
  ams_cell_voltages1/88 -> v4s8_bus/1  "v4s8"
  ams_cell_voltages1/89 -> v10s8_bus/1  "v10s8"
  ams_cell_voltages1/90 -> v4s9_bus/1  "v4s9"
  ams_cell_voltages1/91 -> v10s9_bus/1  "v10s9"
  ams_cell_voltages1/92 -> v4s10_bus/1  "v4s10"
  ams_cell_voltages1/93 -> v10s10_bus/1  "v10s10"
  ams_cell_voltages1/94 -> v4s11_bus/1  "v4s11"
  ams_cell_voltages1/95 -> v10s11_bus/1  "v10s11"
  ams_cell_voltages1/96 -> v4s12_bus/1  "v4s12"
  ams_cell_voltages1/97 -> v10s12_bus/1  "v10s12"
  ams_cell_voltages1/98 -> v5s1_bus/1  "v5s1"
  ams_cell_voltages1/99 -> v11s1_bus/1  "v11s1"
  ams_cell_voltages1/100 -> v5s2_bus/1  "v5s2"
  ams_cell_voltages1/101 -> v5s3_bus/1  "v5s3"
  ams_cell_voltages1/102 -> v11s3_bus/1  "v11s3"
  ams_cell_voltages1/103 -> v5s4_bus/1  "v5s4"
  ams_cell_voltages1/104 -> v5s5_bus/1  "v5s5"
  ams_cell_voltages1/105 -> v11s5_bus/1  "v11s5"
  ams_cell_voltages1/106 -> v5s6_bus/1  "v5s6"
  ams_cell_voltages1/107 -> v5s7_bus/1  "v5s7"
  ams_cell_voltages1/108 -> v11s7_bus/1  "v11s7"
  ams_cell_voltages1/109 -> v5s8_bus/1  "v5s8"
  ams_cell_voltages1/110 -> v5s9_bus/1  "v5s9"
  ams_cell_voltages1/111 -> v11s9_bus/1  "v11s9"
  ams_cell_voltages1/112 -> v5s10_bus/1  "v5s10"
  ams_cell_voltages1/113 -> v5s11_bus/1  "v5s11"
  ams_cell_voltages1/114 -> v11s11_bus/1  "v11s11"
  ams_cell_voltages1/115 -> v5s12_bus/1  "v5s12"
  ams_cell_voltages1/116 -> v6s1_bus/1  "v6s1"
  ams_cell_voltages1/117 -> v6s2_bus/1  "v6s2"
  ams_cell_voltages1/118 -> v6s3_bus/1  "v6s3"
  ams_cell_voltages1/119 -> v6s4_bus/1  "v6s4"
  ams_cell_voltages1/120 -> v6s5_bus/1  "v6s5"
  ams_cell_voltages1/121 -> v6s6_bus/1  "v6s6"
  ams_cell_voltages1/122 -> v6s7_bus/1  "v6s7"
  ams_cell_voltages1/123 -> v6s8_bus/1  "v6s8"
  ams_cell_voltages1/124 -> v6s9_bus/1  "v6s9"
  ams_cell_voltages1/125 -> v6s10_bus/1  "v6s10"
  ams_cell_voltages1/126 -> v6s11_bus/1  "v6s11"
  ams_cell_voltages1/127 -> v6s12_bus/1  "v6s12"
